simulink model "WoundRotorIMWithClosedLoop"  (R2015a)
settings: Solver=ode45  StartTime=0.0  StopTime=5  RelTol=1e-3
libraries: powerlib x9, simulink x2
settings Model: Creator=Soham Roy  LastModifiedBy=Soham Roy

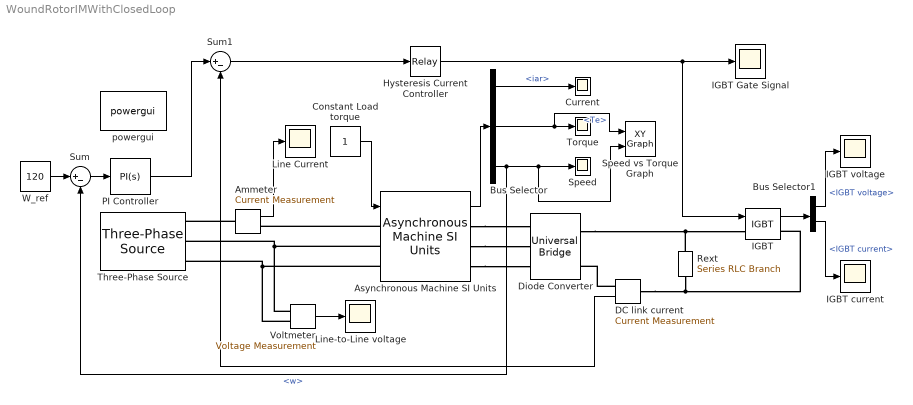
== system WoundRotorIMWithClosedLoop ==
  Ammeter : powerlib/Measurements/Current Measurement  PhasorSimulation=off  OutputType=Complex  PSBequivalent=0
  Asynchronous Machine SI Units : powerlib/Machines/Asynchronous Machine SI Units  RotorType=Wound  PresetModel=No  MechanicalLoad=Torque Tm  ShowDetailedParameters=on  ReferenceFrame=Stationary  Units=SI  MeasurementBus=on  NominalParameters=[2200 400 50]  Stator=[8 0.00203822]  Rotor=[1 0.00203822]  Cage1=[0.4155 0.002066]  Cage2=[0.4168 0.0003495]  Lm=0.0955414  Mechanical=[0.09 0 2]  PolePairs=2  InitialConditions=[1 0 0 0 0 0 0 0]  SimulateSaturation=off  Saturation=[14.03593122, 27.81365428, 53.79336849, 72.68890987, 97.98006896, 148.6815601, 215.7428561, 302.9841135, 428.7778367 ; 230, 322, 414, 460, 506, 552, 598, 644, 690]  LoadFlowParameters=1492000  TsPowergui=0  TsBlock=-1  IterativeModel=Trapezoidal non iterative  Pmec=2200
  Bus Selector : BusSelector  OutputSignals=iar,Te,w
  Bus Selector1 : BusSelector  OutputSignals=IGBT voltage,IGBT current
  Constant Load torque : Constant
  Current : Scope
      settings: YMin=-100  YMax=100
  DC link current : powerlib/Measurements/Current Measurement  PhasorSimulation=off  OutputType=Complex  PSBequivalent=0
  Diode Converter : powerlib/Power Electronics/Universal Bridge  Arms=3  SnubberResistance=1e5  SnubberCapacitance=inf  Device=Diodes  Ron=1e-3  Lon=0  ForwardVoltages="[  0  0  ]"  ForwardVoltage=0  GTOparameters=[ 10e-6 , 20e-6 ]  IGBTparameters=[ 1e-6 , 2e-6 ]  Measurements=None  Measurements_2=None  converterType=Rectifier
  Hysteresis Current Controller : Relay  OnSwitchValue=100  OffSwitchValue=-100
  IGBT : powerlib/Power Electronics/IGBT  Ron=0.001  Lon=0  Vf=1  Tf=1e-6  Tt=2e-6  IC=0  Rs=1e5  Cs=inf  Measurements=on
  IGBT Gate Signal : Scope
      settings: YMin=0.95  YMax=1.05  SaveName=ScopeData8
  IGBT current : Scope
      settings: SaveName=ScopeData6
  IGBT voltage : Scope
      settings: YMin=2.5  YMax=3.9  SaveName=ScopeData5
  Line Current : Scope
      settings: YMin=0.075  YMax=0.55
  Line-to-Line voltage : Scope
      settings: SaveName=ScopeData4
  PI Controller : simulink/Continuous/PID Controller  Controller=PI  TimeDomain=Continuous-time  SampleTime=-1  IntegratorMethod=Forward Euler  FilterMethod=Forward Euler  Form=Parallel  UseFilter=on  ControllerParametersSource=internal  P=1  I=1  D=0  N=100  InitialConditionSource=internal  InitialConditionForIntegrator=0  InitialConditionForFilter=0  ExternalReset=none  LimitOutput=off  UpperSaturationLimit=inf  LowerSaturationLimit=-inf  LinearizeAsGain=on  AntiWindupMode=none  Kb=1  TrackingMode=off  Kt=1  PParamMin=[]  PParamMax=[]  IParamMin=[]  IParamMax=[]  DParamMin=[]  DParamMax=[]  NParamMin=[]  NParamMax=[]  KbParamMin=[]  KbParamMax=[]  KtParamMin=[]  KtParamMax=[]  POutMin=[]  POutMax=[]  IOutMin=[]  IOutMax=[]  DOutMin=[]  DOutMax=[]  NOutMin=[]  NOutMax=[]  KbOutMin=[]  KbOutMax=[]  KtOutMin=[]  KtOutMax=[]  IntegratorOutMin=[]  IntegratorOutMax=[]  FilterOutMin=[]  FilterOutMax=[]  SumOutMin=[]  SumOutMax=[]  SumI1OutMin=[]  SumI1OutMax=[]  SumI2OutMin=[]  SumI2OutMax=[]  SumI3OutMin=[]  SumI3OutMax=[]  SumDOutMin=[]  SumDOutMax=[]  SaturationOutMin=[]  SaturationOutMax=[]  IntegratorContinuousStateAttributes=''  IntegratorStateMustResolveToSignalObject=off  IntegratorRTWStateStorageClass=Auto  FilterContinuousStateAttributes=''  FilterStateMustResolveToSignalObject=off  FilterRTWStateStorageClass=Auto  DifferentiatorICPrevScaledInput=0  DifferentiatorOutMin=[]  DifferentiatorOutMax=[]
  Rext : powerlib/Elements/Series RLC Branch  LConnTagsString=__new0  RConnTagsString=__new0  BranchType=R  Resistance=10  Inductance=1e-3  SetiL0=off  InitialCurrent=0  Capacitance=1e-6  Setx0=off  InitialVoltage=0  Measurements=None
  Speed : Scope
      settings: YMin=0  YMax=170  SaveName=ScopeData2
  Speed vs Torque Graph : simulink/Sinks/XY Graph  xmin=0  xmax=50  ymin=0  ymax=170  st=-1
  Sum : Sum  Inputs=|+-
  Sum1 : Sum  Inputs=|+-
  Three-Phase Source : powerlib/Electrical Sources/Three-Phase Source  Voltage=400  PhaseAngle=0  Frequency=50  InternalConnection=Yg  SpecifyImpedance=off  Resistance=0  Inductance=0  ShortCircuitLevel=100e6  BaseVoltage=400  XRratio=7  BusType=swing  Pref=0  Qref=0  Qmin=-inf  Qmax=inf
  Torque : Scope
      settings: YMin=-20  YMax=50  SaveName=ScopeData3
  Voltmeter : powerlib/Measurements/Voltage Measurement  PhasorSimulation=off  OutputType=Complex  PSBequivalent=0
  W_ref : Constant  Value=120
  powergui : powerlib/powergui  Priority=1  SimulationMode=Continuous  SolverType=Tustin/Backward Euler (TBE)  SampleTime=50e-6  frequency=60  SPID=on  DisableSnubberDevices=off  DisableRonSwitches=off  DisableVfSwitches=off  SwTol=0  DisplayEquations=off  Interpol=off  methode=off  Ts=100  FunctionMessages=off  echomessages=off  HookPort=off  EnableUseOfTLC=off  x0status=blocks  frequencyindice=50  Pbase=100e6  ErrMax=1e-4  Iterations=50  UnitsV=kV  UnitsW=MW  buscounter=0  RestoreLinks=warning  ResistiveCurrentMeasurement=off  Frange=[0:2:500]  Ylog=off  Xlog=on  ShowGrid=off  save=off  variable=ZData  structure=0  ZoomFFT=off  StartTime=0.0  cycles=1  DisplayStyle=1  fundamental=60  FreqAxis=off  MaxFrequency=1000  frequencyindicesteady=1  RmsSteady=1  display=off
  wires:
  Ammeter/1 -> Line Current/1
  Constant Load torque/1 -> Asynchronous Machine SI Units/1
  Voltmeter/1 -> Line-to-Line voltage/1
  Asynchronous Machine SI Units/1 -> Bus Selector/1
  Bus Selector/1 -> Current/1  "<iar>"
  Bus Selector/2 -> Speed vs Torque Graph/1, Torque/1  "<Te>"
  Bus Selector/3 -> Speed vs Torque Graph/2, Speed/1, Sum/2  "<w>"
  IGBT/1 -> Bus Selector1/1
  W_ref/1 -> Sum/1
  Sum/1 -> PI Controller/1
  Bus Selector1/1 -> IGBT voltage/1  "<IGBT voltage>"
  Bus Selector1/2 -> IGBT current/1  "<IGBT current>"
  PI Controller/1 -> Sum1/1
  DC link current/1 -> Sum1/2
  Sum1/1 -> Hysteresis Current Controller/1
  Hysteresis Current Controller/1 -> IGBT/1, IGBT Gate Signal/1
  connections:
  Three-Phase Source/RConn2 -- Asynchronous Machine SI Units/LConn2 -- Voltmeter/LConn1
  Three-Phase Source/RConn3 -- Asynchronous Machine SI Units/LConn3 -- Voltmeter/LConn2
  IGBT/RConn1 -- Rext/RConn1 -- DC link current/LConn1
  Asynchronous Machine SI Units/RConn2 -- Diode Converter/LConn2
  Asynchronous Machine SI Units/RConn1 -- Diode Converter/LConn1
  Ammeter/LConn1 -- Three-Phase Source/RConn1
  Asynchronous Machine SI Units/RConn3 -- Diode Converter/LConn3
  Asynchronous Machine SI Units/LConn1 -- Ammeter/RConn1
  DC link current/RConn1 -- Diode Converter/RConn2
  Rext/LConn1 -- Diode Converter/RConn1 -- IGBT/LConn1
